simulink model "Utkarsh_2005574_R_W2_P2"  (R2021a)
settings: Solver=VariableStepAuto  StartTime=0.0  StopTime=10.0  RelTol=1e-3
PostLoadFcn:
  | be=2;
  | bv=1;
  | Ie=1;
  | Iv=5;
  | muk=1;
  | mus=1.5;
  | R=1;
InitFcn:
  | be=2;
  | bv=1;
  | Ie=1;
  | Iv=5;
  | muk=1;
  | mus=1.5;
  | R=1;
settings Model: Creator=Utkarsh Anand  LastModifiedBy=Utkarsh Anand

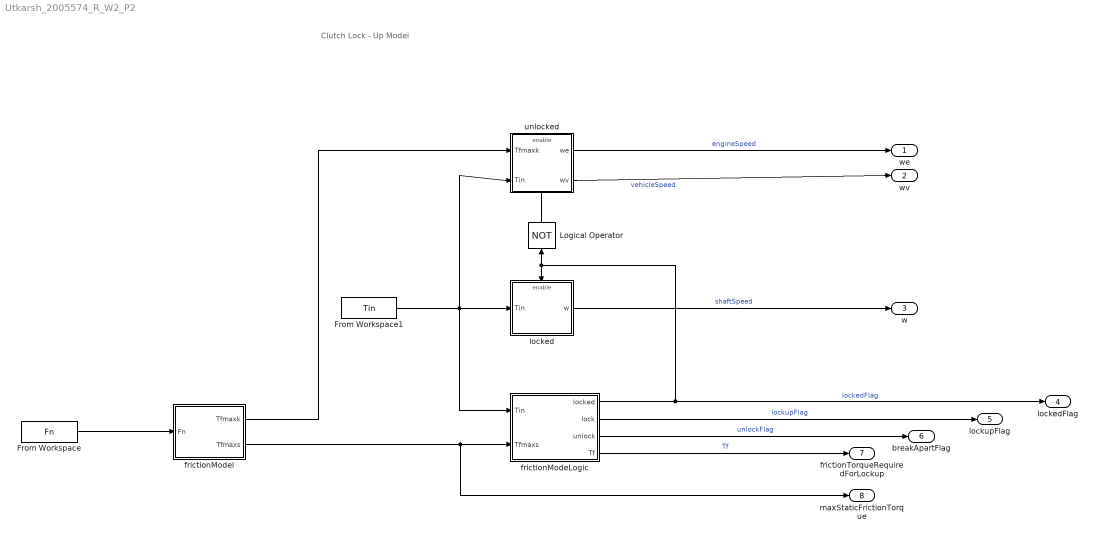
== system Utkarsh_2005574_R_W2_P2 ==
  note: Clutch Lock - Up Model
  From Workspace : FromWorkspace  VariableName=Fn
  From Workspace1 : FromWorkspace  VariableName=Tin
  Logical Operator : Logic  Operator=NOT  IconShape=distinctive  AllPortsSameDT=off  OutDataTypeStr=boolean
  frictionModeLogic : Subsystem
  frictionModel : Subsystem
  locked : Subsystem
  unlocked : Subsystem
  we : Outport
  wv : Outport  Port=2
  w : Outport  Port=3
  lockedFlag : Outport  Port=4
  lockupFlag : Outport  Port=5
  breakApartFlag : Outport  Port=6
  frictionTorqueRequiredForLockup : Outport  Port=7
  maxStaticFrictionTorque : Outport  Port=8
  wires:
  From Workspace/1 -> frictionModel/1(Fn)
  unlocked/1(we) -> we/1  "engineSpeed"
  unlocked/2(wv) -> wv/1  "vehicleSpeed"
  locked/1(w) -> w/1  "shaftSpeed"
  Logical Operator/1 -> unlocked/Enable
  frictionModel/1(Tfmaxk) -> unlocked/1(Tfmaxk)
  frictionModeLogic/1(locked) -> lockedFlag/1, locked/Enable, Logical Operator/1  "lockedFlag"
  frictionModeLogic/2(lock) -> lockupFlag/1  "lockupFlag"
  frictionModeLogic/3(unlock) -> breakApartFlag/1  "unlockFlag"
  frictionModeLogic/4(Tf) -> frictionTorqueRequiredForLockup/1  "Tf"
  From Workspace1/1 -> locked/1(Tin), frictionModeLogic/1(Tin), unlocked/2(Tin)
  frictionModel/2(Tfmaxs) -> maxStaticFrictionTorque/1, frictionModeLogic/2(Tfmaxs)

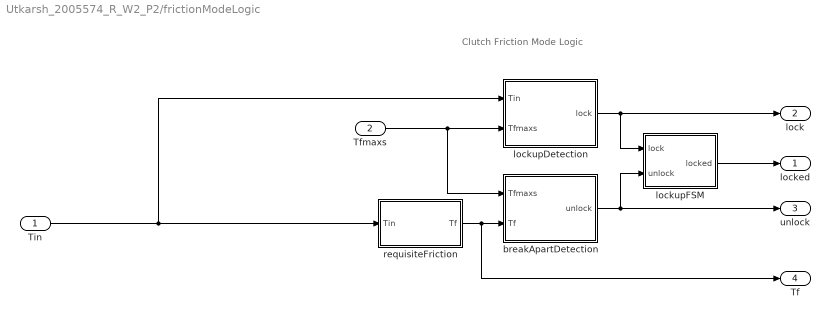
== system Utkarsh_2005574_R_W2_P2/frictionModeLogic ==
  note: Clutch Friction Mode Logic
  Tin : Inport
  Tfmaxs : Inport  Port=2
  breakApartDetection : Subsystem
  lockupDetection : Subsystem
  lockupFSM : Subsystem
  requisiteFriction : Subsystem
  locked : Outport
  lock : Outport  Port=2
  unlock : Outport  Port=3
  Tf : Outport  Port=4
  wires:
  lockupDetection/1(lock) -> lock/1, lockupFSM/1(lock)
  requisiteFriction/1(Tf) -> Tf/1, breakApartDetection/2(Tf)
  breakApartDetection/1(unlock) -> unlock/1, lockupFSM/2(unlock)
  Tin/1 -> lockupDetection/1(Tin), requisiteFriction/1(Tin)
  Tfmaxs/1 -> breakApartDetection/1(Tfmaxs), lockupDetection/2(Tfmaxs)
  lockupFSM/1(locked) -> locked/1

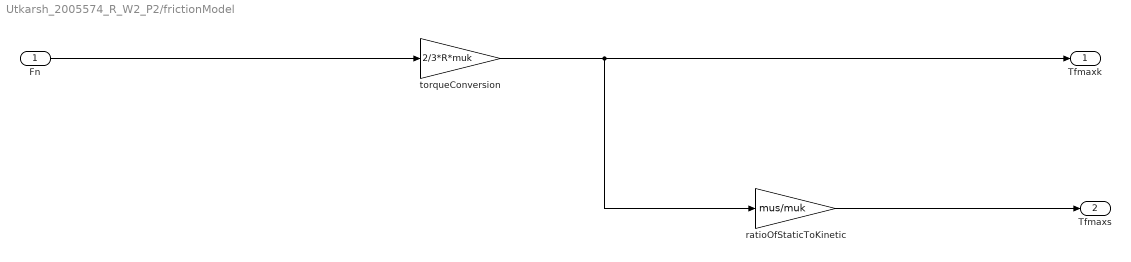
== system Utkarsh_2005574_R_W2_P2/frictionModel ==
  Fn : Inport
  ratioOfStaticToKinetic : Gain  Gain=mus/muk  SaturateOnIntegerOverflow=on  OutDataTypeStr=Inherit: Same as input  ParamDataTypeStr=Inherit: Same as input
  torqueConversion : Gain  Gain=2/3*R*muk  SaturateOnIntegerOverflow=on  OutDataTypeStr=Inherit: Same as input  ParamDataTypeStr=Inherit: Same as input
  Tfmaxk : Outport
  Tfmaxs : Outport  Port=2
  wires:
  torqueConversion/1 -> Tfmaxk/1, ratioOfStaticToKinetic/1
  ratioOfStaticToKinetic/1 -> Tfmaxs/1
  Fn/1 -> torqueConversion/1

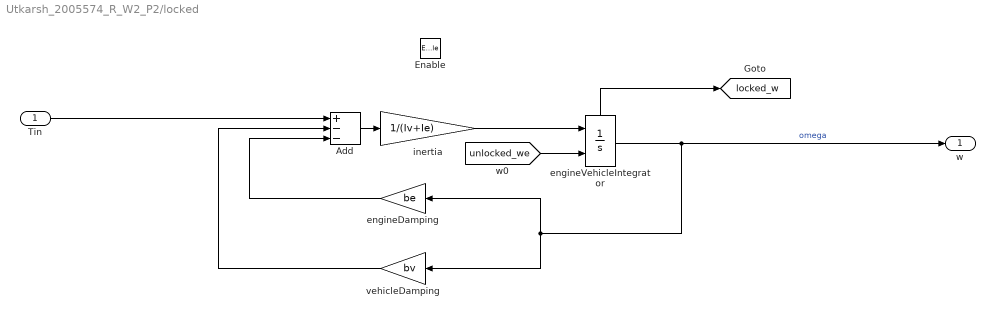
== system Utkarsh_2005574_R_W2_P2/locked ==
  Tin : Inport
  Enable : EnablePort
  Add : Sum  Inputs=+--
  engineDamping : Gain  Gain=be  SaturateOnIntegerOverflow=on  OutDataTypeStr=Inherit: Same as input  ParamDataTypeStr=Inherit: Same as input
  engineVehicleIntegrator : Integrator  InitialConditionSource=external  ShowStatePort=on
  inertia : Gain  Gain=1/(Iv+Ie)  SaturateOnIntegerOverflow=on  OutDataTypeStr=Inherit: Same as input  ParamDataTypeStr=Inherit: Same as input
  vehicleDamping : Gain  Gain=bv  SaturateOnIntegerOverflow=on  OutDataTypeStr=Inherit: Same as input  ParamDataTypeStr=Inherit: Same as input
  w : Outport
  tag scope: locked_w=global
  wires:
  engineVehicleIntegrator/1 -> w/1, engineDamping/1, vehicleDamping/1  "omega"
  [unlocked_we] -> engineVehicleIntegrator/2
  Tin/1 -> Add/1
  vehicleDamping/1 -> Add/2
  inertia/1 -> engineVehicleIntegrator/1
  Add/1 -> inertia/1
  engineVehicleIntegrator/State -> [locked_w]
  engineDamping/1 -> Add/3

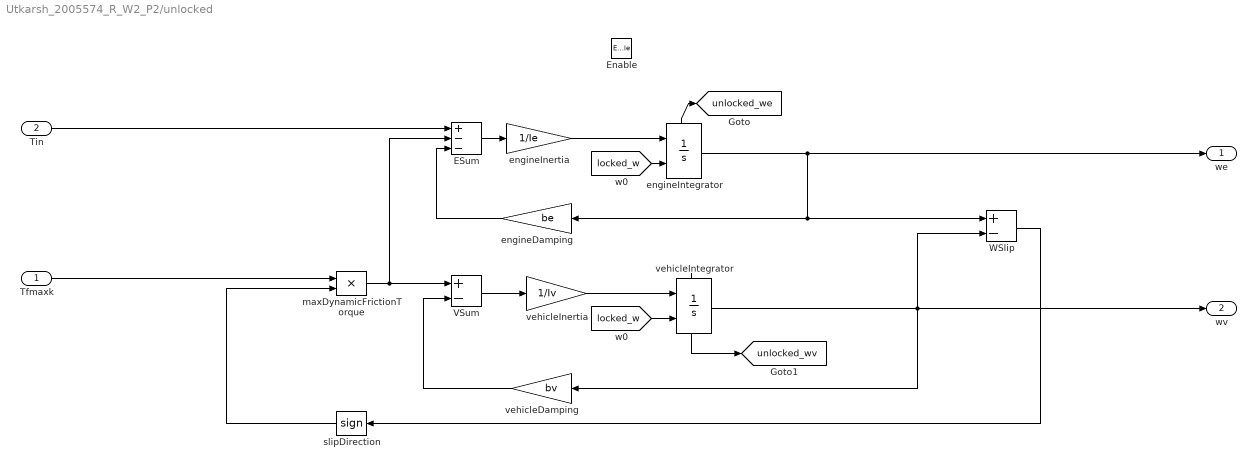
== system Utkarsh_2005574_R_W2_P2/unlocked ==
  Tfmaxk : Inport
  Tin : Inport  Port=2
  Enable : EnablePort
  ESum : Sum  Inputs=+--
  VSum : Sum  Inputs=+-
  WSlip : Sum  Inputs=+-
  engineDamping : Gain  Gain=be  SaturateOnIntegerOverflow=on  OutDataTypeStr=Inherit: Same as input  ParamDataTypeStr=Inherit: Same as input
  engineInertia : Gain  Gain=1/Ie  SaturateOnIntegerOverflow=on  OutDataTypeStr=Inherit: Same as input  ParamDataTypeStr=Inherit: Same as input
  engineIntegrator : Integrator  InitialConditionSource=external  ShowStatePort=on
  maxDynamicFrictionTorque : Product  InputSameDT=on  RndMeth=Zero  SaturateOnIntegerOverflow=on  OutDataTypeStr=Inherit: Same as first input
  slipDirection : Signum
  vehicleDamping : Gain  Gain=bv  SaturateOnIntegerOverflow=on  OutDataTypeStr=Inherit: Same as input  ParamDataTypeStr=Inherit: Same as input
  vehicleInertia : Gain  Gain=1/Iv  SaturateOnIntegerOverflow=on  OutDataTypeStr=Inherit: Same as input  ParamDataTypeStr=Inherit: Same as input
  vehicleIntegrator : Integrator  InitialConditionSource=external  ShowStatePort=on
  we : Outport
  wv : Outport  Port=2
  tag scope: unlocked_we=global, unlocked_wv=global
  wires:
  WSlip/1 -> slipDirection/1
  vehicleInertia/1 -> vehicleIntegrator/1
  engineDamping/1 -> ESum/3
  ESum/1 -> engineInertia/1
  slipDirection/1 -> maxDynamicFrictionTorque/2
  [locked_w] -> engineIntegrator/2
  engineIntegrator/1 -> we/1, engineDamping/1, WSlip/1
  vehicleIntegrator/State -> [unlocked_wv]
  engineInertia/1 -> engineIntegrator/1
  maxDynamicFrictionTorque/1 -> ESum/2, VSum/1
  vehicleIntegrator/1 -> wv/1, vehicleDamping/1, WSlip/2
  [locked_w] -> vehicleIntegrator/2
  engineIntegrator/State -> [unlocked_we]
  vehicleDamping/1 -> VSum/2
  VSum/1 -> vehicleInertia/1
  Tin/1 -> ESum/1
  Tfmaxk/1 -> maxDynamicFrictionTorque/1

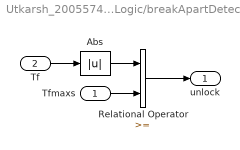
== system Utkarsh_2005574_R_W2_P2/frictionModeLogic/breakApartDetection ==
  Tfmaxs : Inport
  Tf : Inport  Port=2
  Abs : Abs  SaturateOnIntegerOverflow=on
  Relational Operator : RelationalOperator  OutDataTypeStr=boolean  RndMeth=Nearest  InputSameDT=on
  unlock : Outport  InitialOutput=0  VectorParamsAs1DForOutWhenUnconnected=off
  wires:
  Tf/1 -> Abs/1
  Relational Operator/1 -> unlock/1
  Abs/1 -> Relational Operator/1
  Tfmaxs/1 -> Relational Operator/2

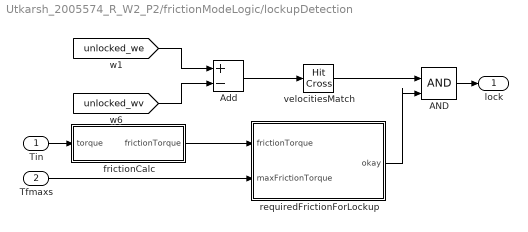
== system Utkarsh_2005574_R_W2_P2/frictionModeLogic/lockupDetection ==
  Tin : Inport
  Tfmaxs : Inport  Port=2
  AND : Logic  IconShape=distinctive  AllPortsSameDT=off  OutDataTypeStr=boolean
  Add : Sum  Inputs=+-
  frictionCalc : Subsystem
  requiredFrictionForLockup : Subsystem
  velocitiesMatch : HitCross
  lock : Outport  InitialOutput=0  VectorParamsAs1DForOutWhenUnconnected=off
  wires:
  frictionCalc/1(frictionTorque) -> requiredFrictionForLockup/1(frictionTorque)
  Tfmaxs/1 -> requiredFrictionForLockup/2(maxFrictionTorque)
  velocitiesMatch/1 -> AND/1
  AND/1 -> lock/1
  requiredFrictionForLockup/1(okay) -> AND/2
  [unlocked_we] -> Add/1
  [unlocked_wv] -> Add/2
  Add/1 -> velocitiesMatch/1
  Tin/1 -> frictionCalc/1(torque)

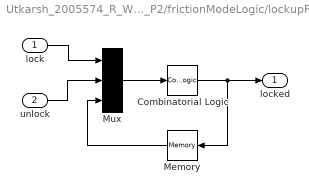
== system Utkarsh_2005574_R_W2_P2/frictionModeLogic/lockupFSM ==
  lock : Inport
  unlock : Inport  Port=2
  Combinatorial Logic : CombinatorialLogic  TruthTable=[0;1;0;0;1;1;1;0]
  Memory : Memory
  Mux : Mux  Inputs=3
  locked : Outport  InitialOutput=0  VectorParamsAs1DForOutWhenUnconnected=off
  wires:
  Memory/1 -> Mux/3
  Combinatorial Logic/1 -> locked/1, Memory/1
  unlock/1 -> Mux/2
  lock/1 -> Mux/1
  Mux/1 -> Combinatorial Logic/1

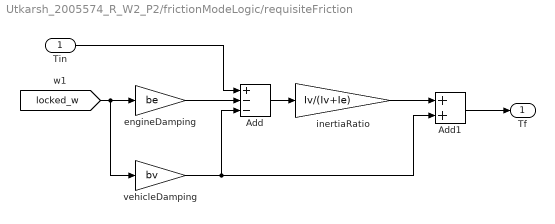
== system Utkarsh_2005574_R_W2_P2/frictionModeLogic/requisiteFriction ==
  Tin : Inport
  Add : Sum  Inputs=+--
  Add1 : Sum
  engineDamping : Gain  Gain=be  SaturateOnIntegerOverflow=on  OutDataTypeStr=Inherit: Same as input  ParamDataTypeStr=Inherit: Same as input
  inertiaRatio : Gain  Gain=Iv/(Iv+Ie)  SaturateOnIntegerOverflow=on  OutDataTypeStr=Inherit: Same as input  ParamDataTypeStr=Inherit: Same as input
  vehicleDamping : Gain  Gain=bv  SaturateOnIntegerOverflow=on  OutDataTypeStr=Inherit: Same as input  ParamDataTypeStr=Inherit: Same as input
  Tf : Outport  InitialOutput=0  VectorParamsAs1DForOutWhenUnconnected=off
  wires:
  [locked_w] -> vehicleDamping/1, engineDamping/1
  engineDamping/1 -> Add/2
  vehicleDamping/1 -> Add1/2, Add/3
  Add/1 -> inertiaRatio/1
  Tin/1 -> Add/1
  inertiaRatio/1 -> Add1/1
  Add1/1 -> Tf/1

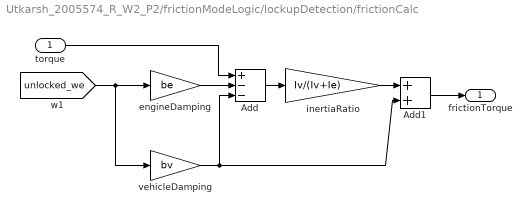
== system Utkarsh_2005574_R_W2_P2/frictionModeLogic/lockupDetection/frictionCalc ==
  torque : Inport
  Add : Sum  Inputs=+--
  Add1 : Sum
  engineDamping : Gain  Gain=be  SaturateOnIntegerOverflow=on  OutDataTypeStr=Inherit: Same as input  ParamDataTypeStr=Inherit: Same as input
  inertiaRatio : Gain  Gain=Iv/(Iv+Ie)  SaturateOnIntegerOverflow=on  OutDataTypeStr=Inherit: Same as input  ParamDataTypeStr=Inherit: Same as input
  vehicleDamping : Gain  Gain=bv  SaturateOnIntegerOverflow=on  OutDataTypeStr=Inherit: Same as input  ParamDataTypeStr=Inherit: Same as input
  frictionTorque : Outport  InitialOutput=0  VectorParamsAs1DForOutWhenUnconnected=off
  wires:
  [unlocked_we] -> engineDamping/1, vehicleDamping/1
  vehicleDamping/1 -> Add/3, Add1/2
  engineDamping/1 -> Add/2
  Add/1 -> inertiaRatio/1
  inertiaRatio/1 -> Add1/1
  Add1/1 -> frictionTorque/1
  torque/1 -> Add/1

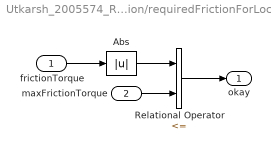
== system Utkarsh_2005574_R_W2_P2/frictionModeLogic/lockupDetection/requiredFrictionForLockup ==
  frictionTorque : Inport
  maxFrictionTorque : Inport  Port=2
  Abs : Abs  SaturateOnIntegerOverflow=on
  Relational Operator : RelationalOperator  Operator=<=  OutDataTypeStr=boolean  RndMeth=Nearest  InputSameDT=on
  okay : Outport  InitialOutput=0  VectorParamsAs1DForOutWhenUnconnected=off
  wires:
  frictionTorque/1 -> Abs/1
  Relational Operator/1 -> okay/1
  Abs/1 -> Relational Operator/1
  maxFrictionTorque/1 -> Relational Operator/2
